simulink model "mmc_model"  (R2023b)
settings: Solver=VariableStepAuto  StartTime=0.0  StopTime=simulation.tsim  RelTol=1e-3
values from neighbouring files (symbols this model uses):
  ab0_to_cell = inv(cell_to_2ab0)    [init_mmc.m]
  cell_to_2ab0 = kron(abc_to_ab0, abc_to_ab0)    [init_mmc.m]
  grid_to_cell = kron(eye(3), ones(3, 1))    [init_mmc.m]
  J = [0 -1; 1 0]    [init_mmc.m]
  machine_to_cell = kron(ones(3, 1), eye(3))    [init_mmc.m]
  volt_to_cell = [      [          1 0 0 0 0 0 ... (first row only)    [init_mmc.m]
undefined symbols (not defined in the file or in its folder): avi, clc, cpu, ctrl, currentControl, DiscIntNeverNeededParam, gfl, grid, load2, loadStep, machine, mmc, pq_ctrl, simulation, soa, stiffGrid, sync, testScenario
libraries: library x17, spsThreePhaseSeriesRLCBranchLib x16, eeGeneralControl x15, spsControlledVoltageSourceLib x15, simulink x11, spsThreePhaseVIMeasurementLib x10, spsGroundLib x9, eeDiscretePi x8, simulink_extras x8, spsabctodq0Lib x8, spsThreePhaseBreakerLib x7, spsdq0toabcLib x5
(part 2 of 3)

== system mmc_model/Electrical Model/Variant Subsystem ==
  note: 1) Add Subsystem or Model blocks as valid variant choices.
      | 2) You cannot connect blocks at this level. At simulation, connectivity is automatically
      | determined, based on the active variant and port name matching.
  GFL_VSC : Subsystem  VariantControl=machine.grid==2
  GFL_VSC_noDC : Subsystem  VariantControl=machine.grid==4
  infinite_bus : Subsystem  VariantControl=machine.grid==0
  short_circuited : Subsystem  VariantControl=machine.grid==3
  synchronous_machine : Subsystem  VariantControl=machine.grid==1
  A : PMIOPort  Side=Left
  B : PMIOPort  Port=2  Side=Left
  C : PMIOPort  Port=3  Side=Left

== system mmc_model/dq_to_ab_g/Subsystem ==
  dq : Inport  PortDimensions=2
  wt : Inport  Port=2  PortDimensions=1
  Fcn : Fcn  Expr=u[1]*cos(u[3]) - u[2]*sin(u[3])
  Fcn1 : Fcn  Expr=u[1]*sin(u[3]) + u[2]*cos(u[3])
  Mux11 : Mux  Inputs=2
  Mux12 : Mux  Inputs=[2 1]
  Mux13 : Mux  Inputs=[2 1]
  alpha_beta : Outport  InitialOutput=[0,0]  VectorParamsAs1DForOutWhenUnconnected=off
  wires:
  wt/1 -> Mux13/2, Mux12/2
  Fcn1/1 -> Mux11/2
  Mux11/1 -> alpha_beta/1
  dq/1 -> Mux13/1, Mux12/1
  Fcn/1 -> Mux11/1
  Mux12/1 -> Fcn/1
  Mux13/1 -> Fcn1/1

== system mmc_model/dq_to_ab_g/Subsystem1 ==
  dq : Inport  PortDimensions=2
  wt : Inport  Port=2  PortDimensions=1
  Fcn : Fcn  Expr=u[1]*cos(u[3]) - u[2]*sin(u[3])
  Fcn1 : Fcn  Expr=u[1]*sin(u[3]) + u[2]*cos(u[3])
  Mux11 : Mux  Inputs=2
  Mux12 : Mux  Inputs=[2 1]
  Mux13 : Mux  Inputs=[2 1]
  alpha_beta : Outport  InitialOutput=[0,0]  VectorParamsAs1DForOutWhenUnconnected=off
  wires:
  wt/1 -> Mux13/2, Mux12/2
  Fcn1/1 -> Mux11/2
  Mux11/1 -> alpha_beta/1
  dq/1 -> Mux13/1, Mux12/1
  Fcn/1 -> Mux11/1
  Mux12/1 -> Fcn/1
  Mux13/1 -> Fcn1/1

== system mmc_model/dq_to_ab_m/Subsystem ==
  dq : Inport  PortDimensions=2
  wt : Inport  Port=2  PortDimensions=1
  Fcn : Fcn  Expr=u[1]*cos(u[3]) - u[2]*sin(u[3])
  Fcn1 : Fcn  Expr=u[1]*sin(u[3]) + u[2]*cos(u[3])
  Mux11 : Mux  Inputs=2
  Mux12 : Mux  Inputs=[2 1]
  Mux13 : Mux  Inputs=[2 1]
  alpha_beta : Outport  InitialOutput=[0,0]  VectorParamsAs1DForOutWhenUnconnected=off
  wires:
  wt/1 -> Mux13/2, Mux12/2
  Fcn1/1 -> Mux11/2
  Mux11/1 -> alpha_beta/1
  dq/1 -> Mux13/1, Mux12/1
  Fcn/1 -> Mux11/1
  Mux12/1 -> Fcn/1
  Mux13/1 -> Fcn1/1

== system mmc_model/dq_to_ab_m/Subsystem1 ==
  dq : Inport  PortDimensions=2
  wt : Inport  Port=2  PortDimensions=1
  Fcn : Fcn  Expr=u[1]*cos(u[3]) - u[2]*sin(u[3])
  Fcn1 : Fcn  Expr=u[1]*sin(u[3]) + u[2]*cos(u[3])
  Mux11 : Mux  Inputs=2
  Mux12 : Mux  Inputs=[2 1]
  Mux13 : Mux  Inputs=[2 1]
  alpha_beta : Outport  InitialOutput=[0,0]  VectorParamsAs1DForOutWhenUnconnected=off
  wires:
  wt/1 -> Mux13/2, Mux12/2
  Fcn1/1 -> Mux11/2
  Mux11/1 -> alpha_beta/1
  dq/1 -> Mux13/1, Mux12/1
  Fcn/1 -> Mux11/1
  Mux12/1 -> Fcn/1
  Mux13/1 -> Fcn1/1

== system mmc_model/dq_to_ab_ns/Subsystem ==
  dq : Inport  PortDimensions=2
  wt : Inport  Port=2  PortDimensions=1
  Fcn : Fcn  Expr=u[1]*cos(u[3]) - u[2]*sin(u[3])
  Fcn1 : Fcn  Expr=u[1]*sin(u[3]) + u[2]*cos(u[3])
  Mux11 : Mux  Inputs=2
  Mux12 : Mux  Inputs=[2 1]
  Mux13 : Mux  Inputs=[2 1]
  alpha_beta : Outport  InitialOutput=[0,0]  VectorParamsAs1DForOutWhenUnconnected=off
  wires:
  wt/1 -> Mux13/2, Mux12/2
  Fcn1/1 -> Mux11/2
  Mux11/1 -> alpha_beta/1
  dq/1 -> Mux13/1, Mux12/1
  Fcn/1 -> Mux11/1
  Mux12/1 -> Fcn/1
  Mux13/1 -> Fcn1/1

== system mmc_model/dq_to_ab_ns/Subsystem1 ==
  dq : Inport  PortDimensions=2
  wt : Inport  Port=2  PortDimensions=1
  Fcn : Fcn  Expr=u[1]*cos(u[3]) - u[2]*sin(u[3])
  Fcn1 : Fcn  Expr=u[1]*sin(u[3]) + u[2]*cos(u[3])
  Mux11 : Mux  Inputs=2
  Mux12 : Mux  Inputs=[2 1]
  Mux13 : Mux  Inputs=[2 1]
  alpha_beta : Outport  InitialOutput=[0,0]  VectorParamsAs1DForOutWhenUnconnected=off
  wires:
  wt/1 -> Mux13/2, Mux12/2
  Fcn1/1 -> Mux11/2
  Mux11/1 -> alpha_beta/1
  dq/1 -> Mux13/1, Mux12/1
  Fcn/1 -> Mux11/1
  Mux12/1 -> Fcn/1
  Mux13/1 -> Fcn1/1

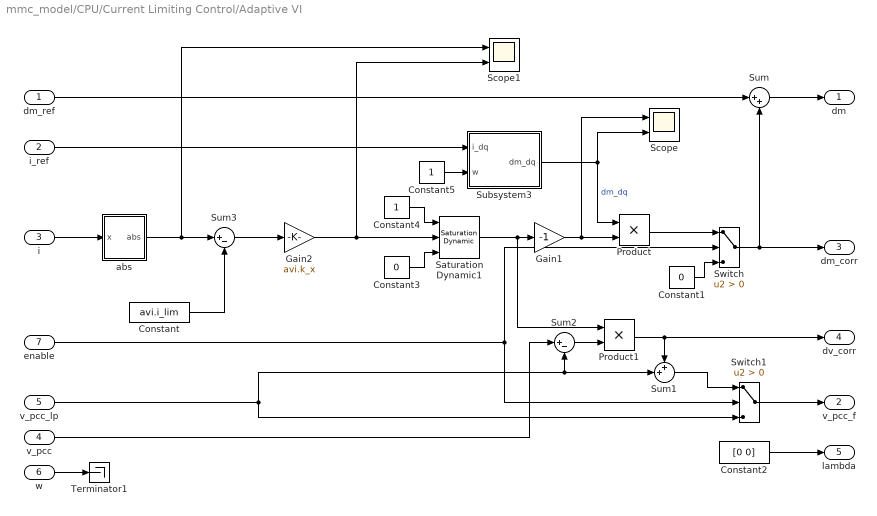
== system mmc_model/CPU/Current Limiting Control/Adaptive VI ==
  dm_ref : Inport
  i_ref : Inport  Port=2
  i : Inport  Port=3
  v_pcc : Inport  Port=4
  v_pcc_lp : Inport  Port=5
  w : Inport  Port=6
  enable : Inport  Port=7
  Constant : Constant  Value=avi.i_lim
  Constant1 : Constant  Value=0
  Constant2 : Constant  Value=[0 0]
  Constant3 : Constant  Value=0
  Constant4 : Constant
  Constant5 : Constant
  Gain1 : Gain  Gain=-1
  Gain2 : Gain  Gain=avi.k_x
  Product : Product
  Product1 : Product
  Saturation Dynamic1 : simulink/Discontinuities/Saturation Dynamic  OutMin=[]  OutMax=[]  OutDataTypeStr=Inherit: Same as second input  OutDataType=fixdt(1, 16)  OutScaling=2^-10  DoSatur=off
  Scope : Scope  NumInputPorts=2
  Scope1 : Scope  NumInputPorts=2
  Subsystem3 : Subsystem
  Sum : Sum  Inputs=|++
  Sum1 : Sum  Inputs=++|
  Sum2 : Sum  Inputs=|+-
  Sum3 : Sum  Inputs=|+-
  Switch : Switch  Criteria=u2 > Threshold  SaturateOnIntegerOverflow=off  InputSameDT=off
  Switch1 : Switch  Criteria=u2 > Threshold  SaturateOnIntegerOverflow=off  InputSameDT=off
  Terminator1 : Terminator
  abs : Subsystem
  dm : Outport
  v_pcc_f : Outport  Port=2
  dm_corr : Outport  Port=3
  dv_corr : Outport  Port=4
  lambda : Outport  Port=5
  wires:
  i/1 -> abs/1(x)
  v_pcc/1 -> Sum2/1
  w/1 -> Terminator1/1
  Constant2/1 -> lambda/1
  Constant/1 -> Sum3/2
  Sum3/1 -> Gain2/1
  abs/1(abs) -> Sum3/1, Scope1/1
  i_ref/1 -> Subsystem3/1(i_dq)
  Subsystem3/1(dm_dq) -> Product/1, Scope/2  "dm_dq"
  dm_ref/1 -> Sum/1
  Sum/1 -> dm/1
  Switch/1 -> Sum/2, dm_corr/1
  enable/1 -> Switch1/2, Switch/2
  Product/1 -> Switch/1
  v_pcc_lp/1 -> Sum2/2, Sum1/2, Switch1/3
  Constant1/1 -> Switch/3
  Constant3/1 -> Saturation Dynamic1/3
  Constant4/1 -> Saturation Dynamic1/1
  Gain2/1 -> Scope1/2, Saturation Dynamic1/2
  Constant5/1 -> Subsystem3/2(w)
  Saturation Dynamic1/1 -> Product1/1, Gain1/1
  Gain1/1 -> Scope/1, Product/2
  Product1/1 -> dv_corr/1, Sum1/1
  Sum1/1 -> Switch1/1
  Sum2/1 -> Product1/2
  Switch1/1 -> v_pcc_f/1

== system mmc_model/CPU/Current Limiting Control/Current Control ==
  dm_ref : Inport
  i_ref : Inport  Port=2
  i : Inport  Port=3
  v_pcc_lp : Inport  Port=4
  enable : Inport  Port=5
  Constant : Constant  Value=currentControl.i_lim
  Constant15 : Constant  Value=0
  Constant2 : Constant  Value=[0 0]
  Logical Operator : Logic  AllPortsSameDT=off  OutDataTypeStr=boolean
  Relay : Relay  OnSwitchValue=0  OffSwitchValue=-0.03
  Scope : Scope  NumInputPorts=2
  Scope1 : Scope
  Sum2 : Sum  Inputs=++|
  Sum3 : Sum  Inputs=|+-
  abs : Subsystem
  iM Control : library/PI Controller  VariantControl=overcurr_ctrl.sel==1  kp=ctrl.machine.ictrl.kp  ti=ctrl.machine.ictrl.ti  Kaw=1
  dm : Outport
  v_pcc_f : Outport  Port=2
  dm_corr : Outport  Port=3
  dv_corr : Outport  Port=4
  lambda : Outport  Port=5
  wires:
  i/1 -> Scope1/1, abs/1(x), iM Control/2
  Constant15/1 -> iM Control/3
  dm_ref/1 -> Sum2/1
  enable/1 -> Logical Operator/2
  Sum2/1 -> dm/1  "dv_m"
  i_ref/1 -> iM Control/1
  iM Control/1 -> dm_corr/1, Sum2/2
  Constant2/1 -> lambda/1, dv_corr/1
  v_pcc_lp/1 -> v_pcc_f/1
  abs/1(abs) -> Sum3/1
  Constant/1 -> Sum3/2
  Relay/1 -> Scope/2, Logical Operator/1
  Logical Operator/1 -> iM Control/4
  Sum3/1 -> Scope/1, Relay/1

== system mmc_model/CPU/Current Limiting Control/Current Limiting Control ==
  dm_ref : Inport
  i_ref : Inport  Port=2
  i : Inport  Port=3
  v_pcc_lp : Inport  Port=4
  w : Inport  Port=5
  enable : Inport  Port=6
  Constant2 : Constant  Value=[0 0]
  Gain : Gain  Gain=1/clc.k_pcc
  Gain1 : Gain  Gain=clc.k_pcc
  Product1 : Product
  SOA_iref : Subsystem
  Scope : Scope  Commented=on  NumInputPorts=3
  Subsystem3 : Subsystem
  Sum2 : Sum  Inputs=|+-
  Sum3 : Sum  Inputs=|-+
  Sum4 : Sum  Inputs=|+-
  Sum5 : Sum  Inputs=|++
  Sum6 : Sum  Inputs=|++
  Terminator1 : Terminator
  dm : Outport
  v_pcc_f : Outport  Port=2
  dm_corr : Outport  Port=3
  dv_corr : Outport  Port=4
  lambda : Outport  Port=5
  wires:
  Constant2/1 -> dv_corr/1, lambda/1
  i/1 -> Sum4/2, Sum5/2, Subsystem3/1(i_dq)
  Sum3/1 -> dm_corr/1
  v_pcc_lp/1 -> v_pcc_f/1
  w/1 -> Subsystem3/2(w)
  Subsystem3/1(dm_dq) -> Sum6/2, Sum2/2  "dm_dq"
  Product1/1 -> Sum3/2, dm/1
  dm_ref/1 -> Sum3/1, Sum2/1
  enable/1 -> Product1/2
  i_ref/1 -> Scope/3
  Sum2/1 -> Gain/1
  Gain/1 -> Sum5/1
  Sum5/1 -> Scope/2, SOA_iref/1(i_ref_dq)
  SOA_iref/1(i_ref_dq_lim) -> Scope/1, Sum4/1  "i_ref_dq"
  Sum4/1 -> Gain1/1
  Gain1/1 -> Sum6/1
  Sum6/1 -> Product1/1

== system mmc_model/CPU/Current Limiting Control/Open Loop ==
  dm_ref : Inport
  v_pcc_lp : Inport  Port=2
  Constant1 : Constant  Value=[0 0]
  dm : Outport
  v_pcc_f : Outport  Port=2
  dm_corr : Outport  Port=3
  dv_corr : Outport  Port=4
  lambda : Outport  Port=5
  wires:
  dm_ref/1 -> dm/1  "dv_m"
  v_pcc_lp/1 -> v_pcc_f/1
  Constant1/1 -> lambda/1, dv_corr/1, dm_corr/1

== system mmc_model/CPU/Current Limiting Control/Safety Filter ==
  dm_ref : Inport
  i_ref : Inport  Port=2
  i : Inport  Port=3
  v_pcc : Inport  Port=4
  enable : Inport  Port=5
  i0 : Inport  Port=6
  v_pcc_lp : Inport  Port=7
  MATLAB Function : MATLAB Function  TreatAsAtomicUnit=on
  Mux : Mux  Inputs=[2 2 2 2 1 1]
  Reshape{,1..3} (4 alike) : Reshape  OutputDimensionality=Customize  OutputDimensions=[2,1]
  Reshape4 : Reshape  OutputDimensionality=Customize  OutputDimensions=[2]
  Reshape5 : Reshape  OutputDimensionality=Customize  OutputDimensions=[2]
  Reshape8 : Reshape  OutputDimensionality=Customize  OutputDimensions=[2]
  Sum : Sum  Inputs=|-+
  correction : Subsystem
  dm : Outport
  v_pcc_f : Outport  Port=2
  dm_corr : Outport  Port=3
  lambda : Outport  Port=4
  wires:
  Reshape1/1 -> Mux/2
  Reshape5/1 -> dm_corr/1
  enable/1 -> Mux/5
  MATLAB Function/2(dm_corr) -> Reshape5/1
  MATLAB Function/1(dm) -> Reshape4/1
  Reshape2/1 -> Mux/3
  dm_ref/1 -> Reshape/1
  Reshape/1 -> Mux/1
  i/1 -> Reshape2/1
  Reshape3/1 -> Mux/4
  Mux/1 -> MATLAB Function/1(u)
  Reshape8/1 -> lambda/1
  MATLAB Function/3(lambda) -> Reshape8/1
  i_ref/1 -> Reshape1/1
  i0/1 -> Mux/6
  Sum/1 -> Reshape3/1
  v_pcc_lp/1 -> v_pcc_f/1, Sum/2
  Reshape4/1 -> dm/1
  v_pcc/1 -> Sum/1

== system mmc_model/CPU/Current Limiting Control/Safety Filter B only ==
  dm_ref : Inport
  i_ref : Inport  Port=2
  i : Inport  Port=3
  v_pcc : Inport  Port=4
  enable : Inport  Port=5
  i0 : Inport  Port=6
  v_pcc_lp : Inport  Port=7
  MATLAB Function : MATLAB Function  TreatAsAtomicUnit=on
  Mux : Mux  Inputs=[2 2 2 2 1 1]
  Reshape{,1..3} (4 alike) : Reshape  OutputDimensionality=Customize  OutputDimensions=[2,1]
  Reshape4 : Reshape  OutputDimensionality=Customize  OutputDimensions=[2]
  Reshape5 : Reshape  OutputDimensionality=Customize  OutputDimensions=[2]
  Reshape8 : Reshape  OutputDimensionality=Customize  OutputDimensions=[2]
  Sum : Sum  Inputs=|-+
  dm : Outport
  v_pcc_f : Outport  Port=2
  dm_corr : Outport  Port=3
  lambda : Outport  Port=4
  wires:
  Reshape1/1 -> Mux/2
  Reshape5/1 -> dm_corr/1
  enable/1 -> Mux/5
  MATLAB Function/2(dm_corr) -> Reshape5/1
  MATLAB Function/1(dm) -> Reshape4/1
  Reshape2/1 -> Mux/3
  dm_ref/1 -> Reshape/1
  Reshape/1 -> Mux/1
  i/1 -> Reshape2/1
  Reshape3/1 -> Mux/4
  Mux/1 -> MATLAB Function/1(u)
  Reshape8/1 -> lambda/1
  MATLAB Function/3(lambda) -> Reshape8/1
  i_ref/1 -> Reshape1/1
  i0/1 -> Mux/6
  Sum/1 -> Reshape3/1
  v_pcc/1 -> Sum/1
  v_pcc_lp/1 -> v_pcc_f/1, Sum/2
  Reshape4/1 -> dm/1

== system mmc_model/CPU/GFM Control/EDPC ==
  pq_ref : Inport
  pq : Inport  Port=2
  v_pcc_abs : Inport  Port=3
  antiwindup : Inport  Port=4
  enable : Inport  Port=5
  Complex to Real-Imag : ComplexToRealImag
  Constant : Constant
  Demux2 : Demux  Outputs=2
  Demux3 : Demux  Outputs=2
  Magnitude-Angle to Complex : MagnitudeAngleToComplex
  Mux1 : Mux  Inputs=2
  NOT1 : Logic  Operator=NOT  IconShape=distinctive  AllPortsSameDT=off  OutDataTypeStr=boolean
  PCtrl : eeDiscretePi/Discrete PI Controller  Kp=pq_ctrl.kp*machine.tr.l  Ki=pq_ctrl.ki*machine.tr.l  Kaw=1000  x0=0  Ts=-1
      settings: LibrarySourceBlock=ee_sl_lib/General Control/Discrete PI Controller
  Product1 : Product
  Product2 : Product
  QCtrl : eeDiscretePi/Discrete PI Controller  Kp=pq_ctrl.kp  Ki=pq_ctrl.ki  Kaw=1000  x0=0  Ts=-1
      settings: LibrarySourceBlock=ee_sl_lib/General Control/Discrete PI Controller
  Saturation : Saturate  UpperLimit=pi/3  LowerLimit=-pi/3
  Scope : Scope  Commented=on
  Sum : Sum  Inputs=|++
  Sum1 : Sum  Inputs=-|+
  Sum2 : Sum  Inputs=|++
  Sum4 : Sum  Inputs=|+-
  abs_phi1 : Scope  Commented=on  NumInputPorts=2
  uQ Droop2 : Gain  Gain=-1
  m : Outport
  wires:
  Sum4/1 -> Demux3/1
  NOT1/1 -> QCtrl/3, PCtrl/3
  pq/1 -> Sum4/2
  Magnitude-Angle to Complex/1 -> Complex to Real-Imag/1
  Complex to Real-Imag/1 -> Mux1/1
  Complex to Real-Imag/2 -> Mux1/2
  Sum2/1 -> Magnitude-Angle to Complex/1
  Product2/1 -> Magnitude-Angle to Complex/2
  Constant/1 -> Sum2/2
  enable/1 -> Product2/1, Product1/1, NOT1/1
  Mux1/1 -> m/1
  antiwindup/1 -> Demux2/1
  PCtrl/1 -> Sum1/1, Saturation/1
  Product1/1 -> Sum2/1
  Demux3/1 -> PCtrl/1
  pq_ref/1 -> Sum4/1
  Demux3/2 -> QCtrl/1
  Saturation/1 -> Sum1/2, abs_phi1/1, Product2/2
  QCtrl/1 -> uQ Droop2/1
  uQ Droop2/1 -> Product1/2, abs_phi1/2
  v_pcc_abs/1 -> Scope/1
  Demux2/2 -> QCtrl/2
  Demux2/1 -> Sum/1
  Sum1/1 -> Sum/2
  Sum/1 -> PCtrl/2

== system mmc_model/CPU/GFM Control/EDPC (modified) ==
  pq_ref : Inport
  pq : Inport  Port=2
  w : Inport  Port=3
  v_pcc_lp : Inport  Port=4
  antiwindup : Inport  Port=5
  enable : Inport  Port=6
  NOT1 : Logic  Operator=NOT  IconShape=distinctive  AllPortsSameDT=off  OutDataTypeStr=boolean
  PQCtrl : eeDiscretePi/Discrete PI Controller  Kp=pq_ctrl.kp  Ki=pq_ctrl.ki  Kaw=1000  x0=0  Ts=-1
      settings: LibrarySourceBlock=ee_sl_lib/General Control/Discrete PI Controller
  Product1 : Product
  Sum2 : Sum  Inputs=|++
  Sum4 : Sum  Inputs=|+-
  Z : Subsystem
  m : Outport
  wires:
  PQCtrl/1 -> Product1/1  "i_ref_dq"
  pq_ref/1 -> Sum4/1  "PQ_ref"
  Sum4/1 -> PQCtrl/1
  NOT1/1 -> PQCtrl/3
  enable/1 -> [enable]
  [enable] -> NOT1/1
  [enable] -> Product1/2
  pq/1 -> Sum4/2
  [w] -> Z/2(w)
  Z/1(dm_dq) -> Sum2/1  "dv_m_ref"
  Product1/1 -> Z/1(i_dq)  "i_ref_dq"
  antiwindup/1 -> PQCtrl/2
  v_pcc_lp/1 -> Sum2/2
  Sum2/1 -> m/1
  w/1 -> [w]

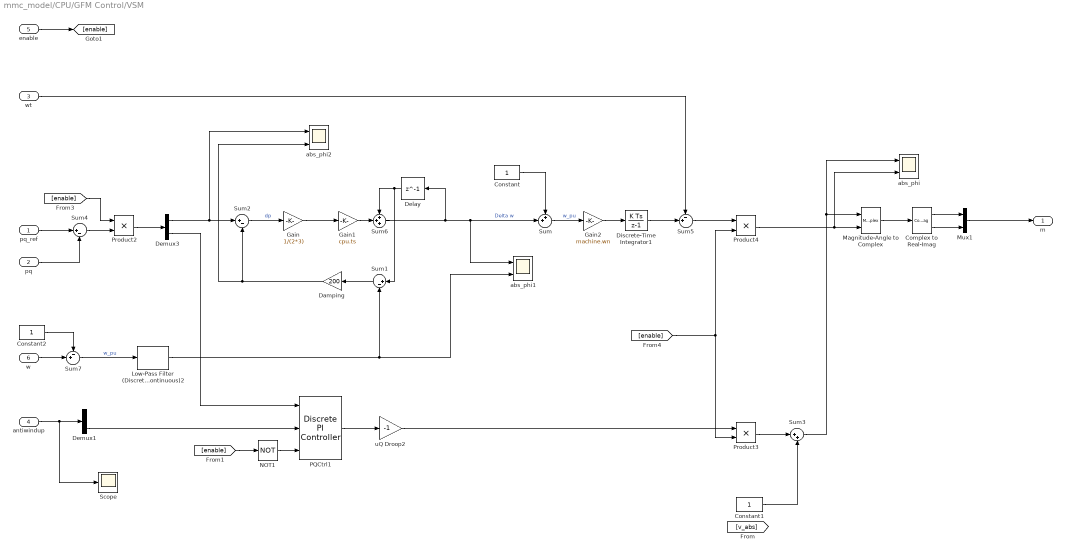
== system mmc_model/CPU/GFM Control/VSM ==
  pq_ref : Inport
  pq : Inport  Port=2
  wt : Inport  Port=3
  antiwindup : Inport  Port=4
  enable : Inport  Port=5
  w : Inport  Port=6
  Complex to Real-Imag : ComplexToRealImag
  Constant : Constant
  Constant1 : Constant
  Constant2 : Constant
  Damping : Gain  Gain=200
  Delay : Delay  DelayLength=1  InitialCondition=0
  Demux1 : Demux  Outputs=2
  Demux3 : Demux  Outputs=2
  Discrete-Time Integrator1 : DiscreteIntegrator  SampleTime=-1  ICPrevOutput=DiscIntNeverNeededParam  ICPrevScaledInput=DiscIntNeverNeededParam
  Gain : Gain  Gain=1/(2*3)
  Gain1 : Gain  Gain=cpu.ts
  Gain2 : Gain  Gain=machine.wn
  Low-Pass Filter (Discrete or Continuous)2 : eeGeneralControl/Low-Pass Filter (Discrete or Continuous)  K=1  T=0.1  B=inf  A=-inf  init_option=Inherited from block input  x0=0  Ts=-1
  Magnitude-Angle to Complex : MagnitudeAngleToComplex
  Mux1 : Mux  Inputs=2
  NOT1 : Logic  Operator=NOT  IconShape=distinctive  AllPortsSameDT=off  OutDataTypeStr=boolean
  PQCtrl1 : eeDiscretePi/Discrete PI Controller  Kp=pq_ctrl.kp  Ki=pq_ctrl.ki  Kaw=1000  x0=0  Ts=-1
      settings: LibrarySourceBlock=ee_sl_lib/General Control/Discrete PI Controller
  Product2 : Product
  Product3 : Product
  Product4 : Product
  Scope : Scope
  Sum : Sum  Inputs=++|
  Sum1 : Sum  Inputs=|+-
  Sum2 : Sum  Inputs=|+-
  Sum3 : Sum  Inputs=|++
  Sum4 : Sum  Inputs=|+-
  Sum5 : Sum  Inputs=-+|
  Sum6 : Sum  Inputs=+++
  Sum7 : Sum  Inputs=-+|
  abs_phi : Scope  NumInputPorts=2
  abs_phi1 : Scope  NumInputPorts=2
  abs_phi2 : Scope  NumInputPorts=2
  uQ Droop2 : Gain  Gain=-1
  m : Outport
  wires:
  Demux3/1 -> abs_phi2/1, Sum2/1
  enable/1 -> [enable]
  Constant/1 -> Sum/1
  Sum1/1 -> Damping/1
  Gain2/1 -> Discrete-Time Integrator1/1
  Sum/1 -> Gain2/1  "w_pu"
  pq/1 -> Sum4/2
  Product2/1 -> Demux3/1
  antiwindup/1 -> Scope/1, Demux1/1
  Demux3/2 -> PQCtrl1/1
  [enable] -> NOT1/1
  NOT1/1 -> PQCtrl1/3
  PQCtrl1/1 -> uQ Droop2/1
  Product3/1 -> Sum3/1
  Sum3/1 -> Magnitude-Angle to Complex/1, abs_phi/1
  Complex to Real-Imag/2 -> Mux1/2
  Magnitude-Angle to Complex/1 -> Complex to Real-Imag/1
  Complex to Real-Imag/1 -> Mux1/1
  Mux1/1 -> m/1
  [enable] -> Product2/1
  wt/1 -> Sum5/1
  Discrete-Time Integrator1/1 -> Sum5/2
  Product4/1 -> abs_phi/2, Magnitude-Angle to Complex/2
  [enable] -> Product4/2, Product3/2
  uQ Droop2/1 -> Product3/1
  Sum5/1 -> Product4/1
  Demux1/2 -> PQCtrl1/2
  Constant1/1 -> Sum3/2
  pq_ref/1 -> Sum4/1
  Sum4/1 -> Product2/2
  Gain1/1 -> Sum6/2
  Delay/1 -> Sum1/1, Sum6/1
  Sum6/1 -> abs_phi1/1, Sum/2, Delay/1  "Delta w"
  Gain/1 -> Gain1/1
  Damping/1 -> abs_phi2/2, Sum2/2
  w/1 -> Sum7/2
  Sum7/1 -> Low-Pass Filter (Discrete or Continuous)2/1  "w_pu"
  Constant2/1 -> Sum7/1
  Sum2/1 -> Gain/1  "dp"
  Low-Pass Filter (Discrete or Continuous)2/1 -> Sum1/2, abs_phi1/2

== system mmc_model/CPU/SOA/SOA_iref ==
  i_ref_dq : Inport
  i_lim_corr : Inport  Port=2
  Constant6 : Constant  Value=soa.i_lim
  Constant7 : Constant  Value=soa.i_lim
  Demux : Demux  Outputs=2
  Gain7 : Gain  Gain=-1
  Gain9 : Gain  Gain=-1
  Mux : Mux  Inputs=2
  Saturation Dynamic1 : simulink/Discontinuities/Saturation Dynamic  OutMin=[]  OutMax=[]  OutDataTypeStr=Inherit: Same as second input  OutDataType=fixdt(1, 16)  OutScaling=2^-10  DoSatur=off
  Saturation Dynamic2 : simulink/Discontinuities/Saturation Dynamic  OutMin=[]  OutMax=[]  OutDataTypeStr=Inherit: Same as second input  OutDataType=fixdt(1, 16)  OutScaling=2^-10  DoSatur=off
  Sqrt3 : Sqrt
  Square1 : Math  Operator=square
  Square4 : Math  Operator=square
  Sum : Sum  Inputs=-+|
  Sum5 : Sum  Inputs=|-+
  i_ref_dq_lim : Outport
  wires:
  Saturation Dynamic1/1 -> Mux/1, Square4/1
  Sqrt3/1 -> Gain7/1, Saturation Dynamic2/1
  Demux/1 -> Saturation Dynamic1/2
  Square4/1 -> Sum5/1
  Sum5/1 -> Sqrt3/1
  Gain7/1 -> Saturation Dynamic2/3
  i_ref_dq/1 -> Demux/1
  Saturation Dynamic2/1 -> Mux/2  "i_q_ref_soa"
  Mux/1 -> i_ref_dq_lim/1
  Square1/1 -> Sum5/2
  Constant6/1 -> Square1/1
  Gain9/1 -> Saturation Dynamic1/3
  Sum/1 -> Saturation Dynamic1/1, Gain9/1
  Constant7/1 -> Sum/2
  i_lim_corr/1 -> Sum/1
  Demux/2 -> Saturation Dynamic2/2

== system mmc_model/CPU/SOA/Subsystem ==
  In1 : Inport
  i_lim_corr : Inport  Port=2
  Cartesian to Polar1 : simulink_extras/Transformations/Cartesian to Polar
  Constant7 : Constant  Value=soa.i_lim
  Demux1 : Demux  Outputs=2
  Gain1 : Gain  Gain=-1
  Mux1 : Mux  Inputs=2
  Polar to Cartesian1 : simulink_extras/Transformations/Polar to Cartesian
  Saturation : Saturate  UpperLimit=inf  LowerLimit=0
  Saturation Dynamic2 : simulink/Discontinuities/Saturation Dynamic  OutMin=[]  OutMax=[]  OutDataTypeStr=Inherit: Same as second input  OutDataType=fixdt(1, 16)  OutScaling=2^-10  DoSatur=off
  Sum : Sum  Inputs=-+|
  Out1 : Outport
  wires:
  Polar to Cartesian1/2 -> Mux1/2
  In1/1 -> Demux1/1
  Gain1/1 -> Saturation Dynamic2/3
  Demux1/1 -> Cartesian to Polar1/1
  Cartesian to Polar1/1 -> Saturation Dynamic2/2
  Sum/1 -> Saturation/1
  Saturation Dynamic2/1 -> Polar to Cartesian1/1
  Demux1/2 -> Cartesian to Polar1/2
  Polar to Cartesian1/1 -> Mux1/1
  Cartesian to Polar1/2 -> Polar to Cartesian1/2
  Mux1/1 -> Out1/1
  i_lim_corr/1 -> Sum/1
  Constant7/1 -> Sum/2
  Saturation/1 -> Gain1/1, Saturation Dynamic2/1

== system mmc_model/CPU/SOA/Subsystem3 ==
  i_dq : Inport
  w : Inport  Port=2
  Gain : Gain  Gain=J  Multiplication=Matrix(K*u) (u vector)
  Gain1 : Gain  Gain=machine.tr.l
  Gain2 : Gain  Gain=machine.tr.r
  Product : Product
  Sum8 : Sum  Inputs=++|
  dm_dq : Outport
  wires:
  Gain1/1 -> Sum8/2
  Sum8/1 -> dm_dq/1  "dm_dq"
  Product/1 -> Gain/1
  Gain/1 -> Gain1/1  "dm_dq"
  w/1 -> Product/1
  i_dq/1 -> Gain2/1, Product/2
  Gain2/1 -> Sum8/1

== system mmc_model/CPU/SOA/Subsystem4 ==
  x : Inport
  y : Inport  Port=2
  Demux : Demux  Outputs=2
  Demux1 : Demux  Outputs=2
  Mux1 : Mux  Inputs=2
  Mux2 : Mux  Inputs=2
  d : Outport
  q : Outport  Port=2
  wires:
  Mux2/1 -> q/1
  y/1 -> Demux1/1
  Demux/2 -> Mux2/1
  Demux1/2 -> Mux2/2
  Demux/1 -> Mux1/1
  Demux1/1 -> Mux1/2
  Mux1/1 -> d/1
  x/1 -> Demux/1

== system mmc_model/CPU/SOA/Z_inv ==
  v : Inport
  w : Inport  Port=2
  Complex to Real-Imag : ComplexToRealImag
  Constant : Constant  Value=machine.tr.r
  Constant1 : Constant  Value=machine.tr.l
  Demux : Demux  Outputs=2
  Divide : Product  Inputs=**
  Divide1 : Product  Inputs=*/
  Mux : Mux  Inputs=2
  Real-Imag to Complex : RealImagToComplex
  Real-Imag to Complex1 : RealImagToComplex
  i : Outport
  wires:
  Real-Imag to Complex1/1 -> Divide1/1
  Complex to Real-Imag/2 -> Mux/2
  Constant/1 -> Real-Imag to Complex/1
  Divide/1 -> Real-Imag to Complex/2
  Demux/2 -> Real-Imag to Complex1/2
  Real-Imag to Complex/1 -> Divide1/2
  Divide1/1 -> Complex to Real-Imag/1
  Constant1/1 -> Divide/1
  Complex to Real-Imag/1 -> Mux/1
  Demux/1 -> Real-Imag to Complex1/1
  w/1 -> Divide/2
  Mux/1 -> i/1
  v/1 -> Demux/1

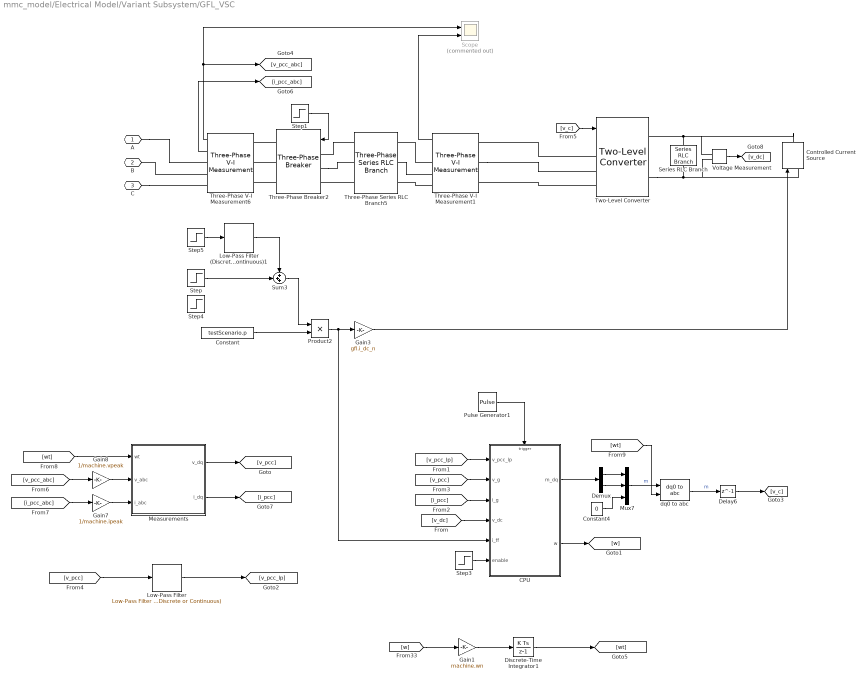
== system mmc_model/Electrical Model/Variant Subsystem/GFL_VSC ==
  CPU : Subsystem
  Constant : Constant  Value=testScenario.p
  Constant4 : Constant  Value=0
  Controlled Current Source : spsControlledCurrentSourceLib/Controlled Current Source  Initialize=on  Source_Type=AC  Amplitude=0  Phase=0  Frequency=0  Measurements=None
  Delay6 : Delay  DelayLength=1  InitialCondition=0  SampleTime=simulation.ts
  Demux : Demux  Outputs=2
  Discrete-Time Integrator1 : DiscreteIntegrator  gainval=1  SampleTime=-1  ICPrevOutput=DiscIntNeverNeededParam  ICPrevScaledInput=DiscIntNeverNeededParam
  Gain1 : Gain  Gain=machine.wn
  Gain3 : Gain  Gain=gfl.i_dc_n
  Gain7 : Gain  Gain=1/machine.ipeak
  Gain8 : Gain  Gain=1/machine.vpeak
  Low-Pass Filter : eeGeneralControl/Low-Pass Filter (Discrete or Continuous)  K=1  T=1/machine.wn*10  B=inf  A=-inf  init_option=Specify as parameter  x0=[1 0 0]  Ts=-1
  Low-Pass Filter (Discrete or Continuous)1 : eeGeneralControl/Low-Pass Filter (Discrete or Continuous)  K=1  T=1e-1  B=inf  A=-inf  init_option=Inherited from block input  x0=0  Ts=-1
  Measurements : Subsystem
  Mux7 : Mux  Inputs=3
  Product2 : Product
  Pulse Generator1 : DiscretePulseGenerator  PulseType=Time based  Period=cpu.ts  PulseWidth=50
  Scope : Scope  Commented=on  NumInputPorts=2
  Series RLC Branch : spsSeriesRLCBranchLib/Series RLC Branch  LConnTagsString=__new0  RConnTagsString=__new0  BranchType=C  Resistance=1  Inductance=1e-3  SetiL0=off  InitialCurrent=0  Capacitance=gfl.c_dc_si  Setx0=on  InitialVoltage=gfl.v_dc  Measurements=None
  Step : Step  Time=loadStep.stepDown  After=-1
  Step1 : Step  Time=gfl.breaker_close
  Step3 : Step  Time=ctrl.grid.ictrl.enable
  Step4 : Step  Time=loadStep.stepUp
  Step5 : Step  Time=gfl.ref_step
  Sum3 : Sum  Inputs=+++
  Three-Phase Series RLC Branch5 : spsThreePhaseSeriesRLCBranchLib/Three-Phase Series RLC Branch  LConnTagsString=A|B|C  RConnTagsString=A|B|C  BranchType=RL  Resistance=gfl.tr.r_si  Inductance=gfl.tr.l_si  Capacitance=1e-6  Measurements=None
  Three-Phase V-I Measurement1 : spsThreePhaseVIMeasurementLib/Three-Phase V-I Measurement  VoltageMeasurement=phase-to-ground  SetLabelV=off  LabelV=Vabc  Vpu=off  VpuLL=off  CurrentMeasurement=yes  SetLabelI=off  LabelI=Iabc  Ipu=off  Pbase=100e6  Vbase=500e3  OutputType=Complex  PhasorSimulation=off  PSBequivalent=0
  Three-Phase V-I Measurement6 : spsThreePhaseVIMeasurementLib/Three-Phase V-I Measurement  VoltageMeasurement=phase-to-ground  SetLabelV=off  LabelV=Vabc  Vpu=off  VpuLL=off  CurrentMeasurement=yes  SetLabelI=off  LabelI=Iabc  Ipu=off  Pbase=100e6  Vbase=500e3  OutputType=Complex  PhasorSimulation=off  PSBequivalent=0
  Three-Phase Breaker2 : spsThreePhaseBreakerLib/Three-Phase Breaker  InitialState=open  SwitchA=on  SwitchB=on  SwitchC=on  SwitchTimes=[machine.breaker_close]  External=on  BreakerResistance=0.01  SnubberResistance=1e6  SnubberCapacitance=inf  Measurements=None
  Two-Level Converter : spsTwoLevelConverterLib/Two-Level Converter  ModelType=Average model (Uref-controlled)  Ron=1e-3  Rs=1e6  Cs=inf  Vforward=[0,0]  Ron_Diode=1e-3  Rs_Diode=1e6  Cs_Diode=inf  Vf_Diode=1e-3  Rs_CurrentSource=inf  Ron_ACsource=1e-3
      settings: LibrarySourceBlock=sps_lib/Power Electronics/Two-Level Converter
  Voltage Measurement : spsVoltageMeasurementLib/Voltage Measurement  PhasorSimulation=off  OutputType=Complex  PSBequivalent=0
  dq0 to abc : spsdq0toabcLib/dq0 to abc  Alignment=Aligned with phase A axis
  A : PMIOPort  Side=Left
  B : PMIOPort  Port=2  Side=Left
  C : PMIOPort  Port=3  Side=Left
  wires:
  [v_pcc_abc] -> Gain8/1
  [i_pcc_abc] -> Gain7/1
  [wt] -> Measurements/1(wt)
  Demux/2 -> Mux7/2
  Constant4/1 -> Mux7/3
  Mux7/1 -> dq0 to abc/1  "m"
  Demux/1 -> Mux7/1
  [wt] -> dq0 to abc/2
  CPU/1(m_dq) -> Demux/1
  [i_pcc] -> CPU/3(i_g)
  Pulse Generator1/1 -> CPU/Trigger
  [v_pcc_lp] -> CPU/1(v_pcc_lp)
  Step3/1 -> CPU/6(enable)
  Measurements/2(i_dq) -> [i_pcc]
  Measurements/1(v_dq) -> [v_pcc]
  [v_pcc] -> Low-Pass Filter/1
  Low-Pass Filter/1 -> [v_pcc_lp]
  Gain7/1 -> Measurements/3(i_abc)
  Gain8/1 -> Measurements/2(v_abc)
  CPU/2(w) -> [w]
  [v_pcc] -> CPU/2(v_g)
  [w] -> Gain1/1
  Gain1/1 -> Discrete-Time Integrator1/1
  Discrete-Time Integrator1/1 -> [wt]
  Step1/1 -> Three-Phase Breaker2/1
  Three-Phase V-I Measurement6/1 -> [v_pcc_abc], Scope/1
  Three-Phase V-I Measurement6/2 -> [i_pcc_abc]
  dq0 to abc/1 -> Delay6/1  "m"
  Delay6/1 -> [v_c]
  Voltage Measurement/1 -> [v_dc]
  [v_c] -> Two-Level Converter/1
  [v_dc] -> CPU/4(v_dc)
  Three-Phase V-I Measurement1/1 -> Scope/2
  Low-Pass Filter (Discrete or Continuous)1/1 -> Sum3/1
  Step5/1 -> Low-Pass Filter (Discrete or Continuous)1/1
  Sum3/1 -> Product2/1
  Constant/1 -> Product2/2
  Product2/1 -> CPU/5(i_ff), Gain3/1
  Gain3/1 -> Controlled Current Source/1
  Step/1 -> Sum3/2
  connections:
  Three-Phase Series RLC Branch5/LConn3 -- Three-Phase Breaker2/LConn3
  Three-Phase Breaker2/RConn1 -- Three-Phase V-I Measurement6/LConn1
  Three-Phase Breaker2/RConn2 -- Three-Phase V-I Measurement6/LConn2
  Three-Phase Breaker2/LConn2 -- Three-Phase Series RLC Branch5/LConn2
  Three-Phase Series RLC Branch5/LConn1 -- Three-Phase Breaker2/LConn1
  Three-Phase Breaker2/RConn3 -- Three-Phase V-I Measurement6/LConn3
  A/RConn1 -- Three-Phase V-I Measurement6/RConn1
  Three-Phase V-I Measurement6/RConn2 -- B/RConn1
  C/RConn1 -- Three-Phase V-I Measurement6/RConn3
  Two-Level Converter/LConn1 -- Three-Phase V-I Measurement1/LConn1
  Three-Phase V-I Measurement1/LConn2 -- Two-Level Converter/LConn2
  Two-Level Converter/LConn3 -- Three-Phase V-I Measurement1/LConn3
  Series RLC Branch/LConn1 -- Voltage Measurement/LConn1 -- Controlled Current Source/RConn1 -- Two-Level Converter/RConn1
  Two-Level Converter/RConn2 -- Voltage Measurement/LConn2 -- Controlled Current Source/LConn1 -- Series RLC Branch/RConn1
  Three-Phase V-I Measurement1/RConn1 -- Three-Phase Series RLC Branch5/RConn1
  Three-Phase Series RLC Branch5/RConn2 -- Three-Phase V-I Measurement1/RConn2
  Three-Phase V-I Measurement1/RConn3 -- Three-Phase Series RLC Branch5/RConn3

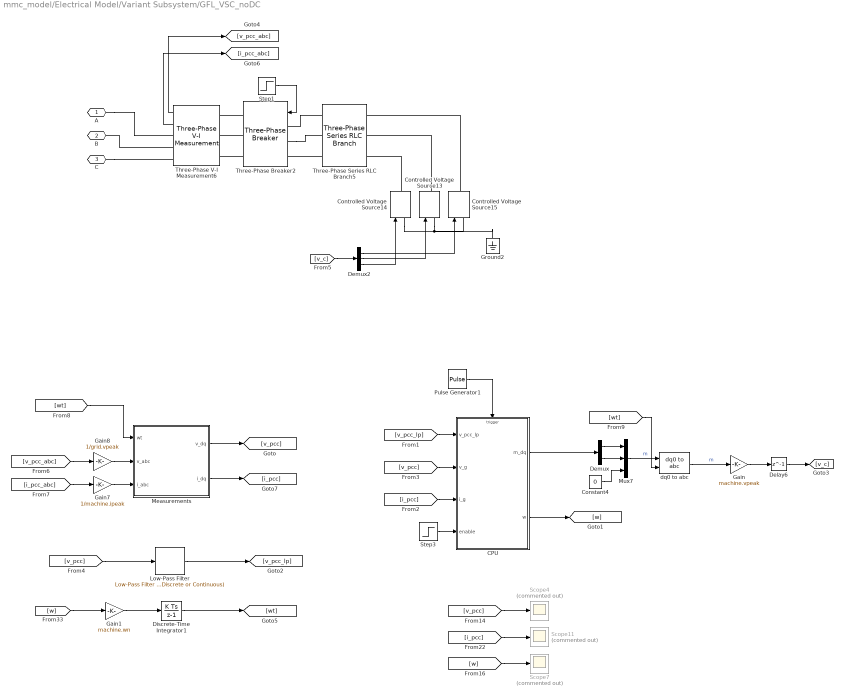
== system mmc_model/Electrical Model/Variant Subsystem/GFL_VSC_noDC ==
  CPU : Subsystem
  Constant4 : Constant  Value=0
  Controlled Voltage Source13 : spsControlledVoltageSourceLib/Controlled Voltage Source  Initialize=on  Source_Type=AC  Amplitude=0  Phase=0  Frequency=0  Measurements=None
  Controlled Voltage Source14 : spsControlledVoltageSourceLib/Controlled Voltage Source  Initialize=on  Source_Type=AC  Amplitude=0  Phase=0  Frequency=0  Measurements=None
  Controlled Voltage Source15 : spsControlledVoltageSourceLib/Controlled Voltage Source  Initialize=on  Source_Type=AC  Amplitude=0  Phase=0  Frequency=0  Measurements=None
  Delay6 : Delay  DelayLength=1  InitialCondition=0  SampleTime=simulation.ts
  Demux : Demux  Outputs=2
  Demux2 : Demux  Outputs=3
  Discrete-Time Integrator1 : DiscreteIntegrator  gainval=1  SampleTime=-1  ICPrevOutput=DiscIntNeverNeededParam  ICPrevScaledInput=DiscIntNeverNeededParam
  Gain : Gain  Gain=machine.vpeak
  Gain1 : Gain  Gain=machine.wn
  Gain7 : Gain  Gain=1/machine.ipeak
  Gain8 : Gain  Gain=1/grid.vpeak
  Ground2 : spsGroundLib/Ground  LConnTagsString=a
  Low-Pass Filter : eeGeneralControl/Low-Pass Filter (Discrete or Continuous)  K=1  T=1/machine.wn*10  B=inf  A=-inf  init_option=Specify as parameter  x0=[1 0 0]  Ts=-1
  Measurements : Subsystem
  Mux7 : Mux  Inputs=3
  Pulse Generator1 : DiscretePulseGenerator  PulseType=Time based  Period=cpu.ts  PulseWidth=50
  Scope11 : Scope  Commented=on
  Scope4 : Scope  Commented=on
  Scope7 : Scope  Commented=on
  Step1 : Step  Time=gfl.breaker_close
  Step3 : Step  Time=gfl.ctrl_enable
  Three-Phase Series RLC Branch5 : spsThreePhaseSeriesRLCBranchLib/Three-Phase Series RLC Branch  LConnTagsString=A|B|C  RConnTagsString=A|B|C  BranchType=RL  Resistance=gfl.tr.r_si  Inductance=gfl.tr.l_si  Capacitance=1e-6  Measurements=None
  Three-Phase V-I Measurement6 : spsThreePhaseVIMeasurementLib/Three-Phase V-I Measurement  VoltageMeasurement=phase-to-ground  SetLabelV=off  LabelV=Vabc  Vpu=off  VpuLL=off  CurrentMeasurement=yes  SetLabelI=off  LabelI=Iabc  Ipu=off  Pbase=100e6  Vbase=500e3  OutputType=Complex  PhasorSimulation=off  PSBequivalent=0
  Three-Phase Breaker2 : spsThreePhaseBreakerLib/Three-Phase Breaker  InitialState=open  SwitchA=on  SwitchB=on  SwitchC=on  SwitchTimes=[machine.breaker_close]  External=on  BreakerResistance=0.01  SnubberResistance=1e6  SnubberCapacitance=inf  Measurements=None
  dq0 to abc : spsdq0toabcLib/dq0 to abc  Alignment=Aligned with phase A axis
  A : PMIOPort  Side=Left
  B : PMIOPort  Port=2  Side=Left
  C : PMIOPort  Port=3  Side=Left
  wires:
  [v_pcc_abc] -> Gain8/1
  [i_pcc_abc] -> Gain7/1
  [wt] -> Measurements/1(wt)
  Demux/2 -> Mux7/2
  Constant4/1 -> Mux7/3
  Mux7/1 -> dq0 to abc/1  "m"
  Demux/1 -> Mux7/1
  [wt] -> dq0 to abc/2
  Gain/1 -> Delay6/1
  CPU/1(m_dq) -> Demux/1
  [i_pcc] -> CPU/3(i_g)
  Pulse Generator1/1 -> CPU/Trigger
  [v_pcc_lp] -> CPU/1(v_pcc_lp)
  Step3/1 -> CPU/4(enable)
  Measurements/2(i_dq) -> [i_pcc]
  Measurements/1(v_dq) -> [v_pcc]
  [v_pcc] -> Low-Pass Filter/1
  Low-Pass Filter/1 -> [v_pcc_lp]
  [w] -> Scope7/1
  [i_pcc] -> Scope11/1
  [v_pcc] -> Scope4/1
  Gain7/1 -> Measurements/3(i_abc)
  Gain8/1 -> Measurements/2(v_abc)
  CPU/2(w) -> [w]
  [v_pcc] -> CPU/2(v_g)
  [w] -> Gain1/1
  Gain1/1 -> Discrete-Time Integrator1/1
  Discrete-Time Integrator1/1 -> [wt]
  Step1/1 -> Three-Phase Breaker2/1
  Demux2/3 -> Controlled Voltage Source14/1
  Demux2/1 -> Controlled Voltage Source15/1
  Demux2/2 -> Controlled Voltage Source13/1
  [v_c] -> Demux2/1
  Three-Phase V-I Measurement6/1 -> [v_pcc_abc]
  Three-Phase V-I Measurement6/2 -> [i_pcc_abc]
  dq0 to abc/1 -> Gain/1  "m"
  Delay6/1 -> [v_c]
  connections:
  Controlled Voltage Source14/LConn1 -- Ground2/LConn1 -- Controlled Voltage Source15/LConn1 -- Controlled Voltage Source13/LConn1
  Three-Phase Series RLC Branch5/LConn3 -- Three-Phase Breaker2/LConn3
  Three-Phase Breaker2/RConn1 -- Three-Phase V-I Measurement6/LConn1
  Three-Phase Breaker2/RConn2 -- Three-Phase V-I Measurement6/LConn2
  Three-Phase Breaker2/LConn2 -- Three-Phase Series RLC Branch5/LConn2
  Controlled Voltage Source15/RConn1 -- Three-Phase Series RLC Branch5/RConn1
  Three-Phase Series RLC Branch5/LConn1 -- Three-Phase Breaker2/LConn1
  Controlled Voltage Source13/RConn1 -- Three-Phase Series RLC Branch5/RConn2
  Three-Phase Breaker2/RConn3 -- Three-Phase V-I Measurement6/LConn3
  Controlled Voltage Source14/RConn1 -- Three-Phase Series RLC Branch5/RConn3
  A/RConn1 -- Three-Phase V-I Measurement6/RConn1
  Three-Phase V-I Measurement6/RConn2 -- B/RConn1
  C/RConn1 -- Three-Phase V-I Measurement6/RConn3

== system mmc_model/Electrical Model/Variant Subsystem/infinite_bus ==
  Controlled Voltage Source13 : spsControlledVoltageSourceLib/Controlled Voltage Source  Initialize=on  Source_Type=AC  Amplitude=0  Phase=0  Frequency=0  Measurements=None
  Controlled Voltage Source14 : spsControlledVoltageSourceLib/Controlled Voltage Source  Initialize=on  Source_Type=AC  Amplitude=0  Phase=0  Frequency=0  Measurements=None
  Controlled Voltage Source15 : spsControlledVoltageSourceLib/Controlled Voltage Source  Initialize=on  Source_Type=AC  Amplitude=0  Phase=0  Frequency=0  Measurements=None
  Demux2 : Demux  Outputs=3
  Ground2 : spsGroundLib/Ground  LConnTagsString=a
  Mux : Mux  Inputs=3
  Sine Wave3 : Sin  Amplitude=stiffGrid.vpeak  Frequency=stiffGrid.w  Phase=pi/2  SampleTime=0
  Sine Wave4 : Sin  Amplitude=stiffGrid.vpeak  Frequency=stiffGrid.w  Phase=pi/2-2*pi/3  SampleTime=0
  Sine Wave5 : Sin  Amplitude=stiffGrid.vpeak  Frequency=stiffGrid.w  Phase=pi/2+2*pi/3  SampleTime=0
  Three-Phase Series RLC Branch5 : spsThreePhaseSeriesRLCBranchLib/Three-Phase Series RLC Branch  LConnTagsString=A|B|C  RConnTagsString=A|B|C  BranchType=RL  Resistance=stiffGrid.r_si  Inductance=stiffGrid.l_si  Capacitance=1e-6  Measurements=None
  A : PMIOPort  Side=Left
  B : PMIOPort  Port=2  Side=Left
  C : PMIOPort  Port=3  Side=Left
  wires:
  Mux/1 -> Demux2/1
  Demux2/2 -> Controlled Voltage Source13/1
  Demux2/1 -> Controlled Voltage Source15/1
  Demux2/3 -> Controlled Voltage Source14/1
  Sine Wave5/1 -> Mux/3
  Sine Wave3/1 -> Mux/1
  Sine Wave4/1 -> Mux/2
  connections:
  Controlled Voltage Source13/LConn1 -- Controlled Voltage Source14/LConn1 -- Ground2/LConn1 -- Controlled Voltage Source15/LConn1
  Controlled Voltage Source13/RConn1 -- Three-Phase Series RLC Branch5/RConn2
  Controlled Voltage Source14/RConn1 -- Three-Phase Series RLC Branch5/RConn3
  Controlled Voltage Source15/RConn1 -- Three-Phase Series RLC Branch5/RConn1
  A/RConn1 -- Three-Phase Series RLC Branch5/LConn1
  B/RConn1 -- Three-Phase Series RLC Branch5/LConn2
  Three-Phase Series RLC Branch5/LConn3 -- C/RConn1

== system mmc_model/Electrical Model/Variant Subsystem/short_circuited ==
  Ground1 : spsGroundLib/Ground  LConnTagsString=a
  Three-Phase Series RLC Branch1 : spsThreePhaseSeriesRLCBranchLib/Three-Phase Series RLC Branch  LConnTagsString=A|B|C  RConnTagsString=A|B|C  BranchType=R  Resistance=100  Inductance=load2.l_si  Capacitance=1e-6  Measurements=None
  Three-Phase Series RLC Branch7 : spsThreePhaseSeriesRLCBranchLib/Three-Phase Series RLC Branch  LConnTagsString=A|B|C  RConnTagsString=A|B|C  BranchType=R  Resistance=100  Inductance=load2.l_si  Capacitance=1e-6  Measurements=None
  Three-Phase Breaker1 : spsThreePhaseBreakerLib/Three-Phase Breaker  InitialState=open  SwitchA=on  SwitchB=on  SwitchC=on  SwitchTimes=[1.4]  External=off  BreakerResistance=0.01  SnubberResistance=1e6  SnubberCapacitance=inf  Measurements=None
  A : PMIOPort  Side=Left
  B : PMIOPort  Port=2  Side=Left
  C : PMIOPort  Port=3  Side=Left
  connections:
  A/RConn1 -- Three-Phase Breaker1/LConn1 -- Three-Phase Series RLC Branch7/LConn1
  B/RConn1 -- Three-Phase Breaker1/LConn2 -- Three-Phase Series RLC Branch7/LConn2
  C/RConn1 -- Three-Phase Breaker1/LConn3 -- Three-Phase Series RLC Branch7/LConn3
  Ground1/LConn1 -- Three-Phase Series RLC Branch7/RConn3 -- Three-Phase Series RLC Branch7/RConn2 -- Three-Phase Series RLC Branch1/RConn2 -- Three-Phase Series RLC Branch1/RConn1 -- Three-Phase Series RLC Branch1/RConn3 -- Three-Phase Series RLC Branch7/RConn1
  Three-Phase Breaker1/RConn1 -- Three-Phase Series RLC Branch1/LConn1
  Three-Phase Breaker1/RConn2 -- Three-Phase Series RLC Branch1/LConn2
  Three-Phase Breaker1/RConn3 -- Three-Phase Series RLC Branch1/LConn3

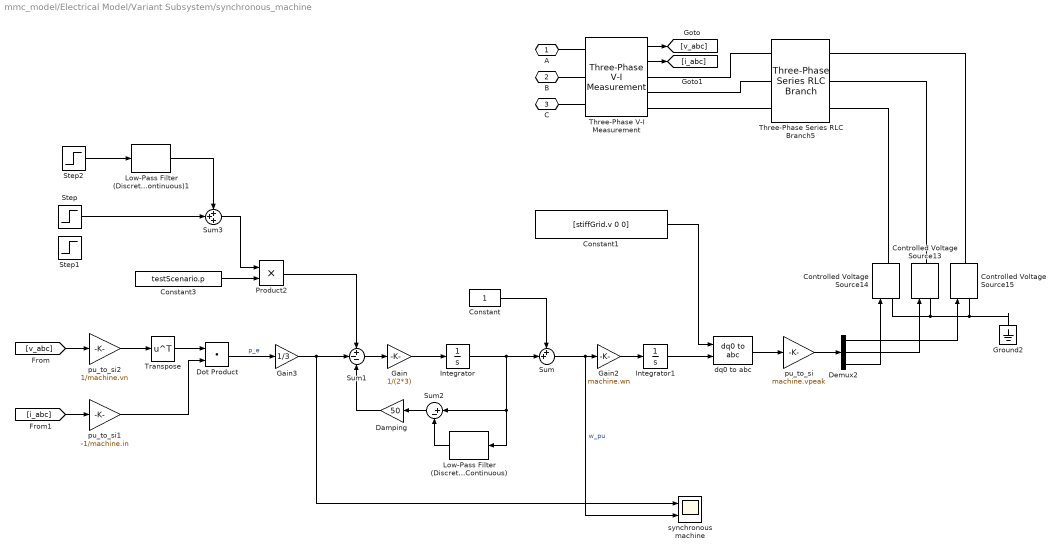
== system mmc_model/Electrical Model/Variant Subsystem/synchronous_machine ==
  Constant : Constant
  Constant1 : Constant  Value=[stiffGrid.v 0 0]
  Constant3 : Constant  Value=testScenario.p
  Controlled Voltage Source13 : spsControlledVoltageSourceLib/Controlled Voltage Source  Initialize=on  Source_Type=AC  Amplitude=0  Phase=0  Frequency=0  Measurements=None
  Controlled Voltage Source14 : spsControlledVoltageSourceLib/Controlled Voltage Source  Initialize=on  Source_Type=AC  Amplitude=0  Phase=0  Frequency=0  Measurements=None
  Controlled Voltage Source15 : spsControlledVoltageSourceLib/Controlled Voltage Source  Initialize=on  Source_Type=AC  Amplitude=0  Phase=0  Frequency=0  Measurements=None
  Damping : Gain  Gain=50
  Demux2 : Demux  Outputs=3
  Dot Product : DotProduct  OutDataTypeStr=Inherit: Inherit via internal rule
  Gain : Gain  Gain=1/(2*3)
  Gain2 : Gain  Gain=machine.wn
  Gain3 : Gain  Gain=1/3
  Ground2 : spsGroundLib/Ground  LConnTagsString=a
  Integrator : Integrator
  Integrator1 : Integrator
  Low-Pass Filter (Discrete or Continuous) : eeGeneralControl/Low-Pass Filter (Discrete or Continuous)  K=1  T=0.1  B=inf  A=-inf  init_option=Inherited from block input  x0=0  Ts=-1
  Low-Pass Filter (Discrete or Continuous)1 : eeGeneralControl/Low-Pass Filter (Discrete or Continuous)  K=1  T=0.1  B=inf  A=-inf  init_option=Inherited from block input  x0=0  Ts=-1
  Product2 : Product
  Step : Step  Time=loadStep.stepDown  After=-1  SampleTime=0
  Step1 : Step  Time=loadStep.stepUp  After=0.8  SampleTime=0
  Step2 : Step  Time=0.3  SampleTime=0
  Sum : Sum  Inputs=++|
  Sum1 : Sum  Inputs=+--
  Sum2 : Sum  Inputs=|+-
  Sum3 : Sum  Inputs=+++
  Three-Phase Series RLC Branch5 : spsThreePhaseSeriesRLCBranchLib/Three-Phase Series RLC Branch  LConnTagsString=A|B|C  RConnTagsString=A|B|C  BranchType=RL  Resistance=machine.tr.r_si  Inductance=machine.tr.l_si  Capacitance=1e-6  Measurements=None
  Three-Phase V-I Measurement : spsThreePhaseVIMeasurementLib/Three-Phase V-I Measurement  VoltageMeasurement=phase-to-ground  SetLabelV=off  LabelV=Vabc  Vpu=off  VpuLL=off  CurrentMeasurement=yes  SetLabelI=off  LabelI=Iabc  Ipu=off  Pbase=100e6  Vbase=500e3  OutputType=Complex  PhasorSimulation=off  PSBequivalent=0
  Transpose : Math  Operator=transpose
  dq0 to abc : spsdq0toabcLib/dq0 to abc  Alignment=Aligned with phase A axis
  pu_to_si : Gain  Gain=machine.vpeak
  pu_to_si1 : Gain  Gain=-1/machine.in
  pu_to_si2 : Gain  Gain=1/machine.vn
  synchronous machine : Scope  NumInputPorts=2
  A : PMIOPort  Side=Left
  B : PMIOPort  Port=2  Side=Left
  C : PMIOPort  Port=3  Side=Left
  wires:
  Demux2/2 -> Controlled Voltage Source13/1
  Demux2/1 -> Controlled Voltage Source15/1
  Demux2/3 -> Controlled Voltage Source14/1
  Transpose/1 -> Dot Product/1
  Dot Product/1 -> Gain3/1  "p_e"
  Gain/1 -> Integrator/1
  Sum1/1 -> Gain/1
  Sum2/1 -> Damping/1
  Low-Pass Filter (Discrete or Continuous)/1 -> Sum2/2
  Constant/1 -> Sum/1
  Sum/1 -> synchronous machine/2, Gain2/1  "w_pu"
  Gain2/1 -> Integrator1/1
  dq0 to abc/1 -> pu_to_si/1
  Integrator1/1 -> dq0 to abc/2
  Constant1/1 -> dq0 to abc/1
  pu_to_si/1 -> Demux2/1
  pu_to_si1/1 -> Dot Product/2
  pu_to_si2/1 -> Transpose/1
  Damping/1 -> Sum1/3
  Three-Phase V-I Measurement/1 -> [v_abc]
  Three-Phase V-I Measurement/2 -> [i_abc]
  [i_abc] -> pu_to_si1/1
  [v_abc] -> pu_to_si2/1
  Gain3/1 -> Sum1/2, synchronous machine/1
  Sum3/1 -> Product2/1
  Constant3/1 -> Product2/2
  Step2/1 -> Low-Pass Filter (Discrete or Continuous)1/1
  Low-Pass Filter (Discrete or Continuous)1/1 -> Sum3/1
  Product2/1 -> Sum1/1
  Integrator/1 -> Sum/2, Sum2/1, Low-Pass Filter (Discrete or Continuous)/1
  Step/1 -> Sum3/2
  connections:
  Ground2/LConn1 -- Controlled Voltage Source15/LConn1 -- Controlled Voltage Source13/LConn1 -- Controlled Voltage Source14/LConn1
  Controlled Voltage Source13/RConn1 -- Three-Phase Series RLC Branch5/RConn2
  Controlled Voltage Source14/RConn1 -- Three-Phase Series RLC Branch5/RConn3
  Controlled Voltage Source15/RConn1 -- Three-Phase Series RLC Branch5/RConn1
  A/RConn1 -- Three-Phase V-I Measurement/LConn1
  B/RConn1 -- Three-Phase V-I Measurement/LConn2
  Three-Phase V-I Measurement/LConn3 -- C/RConn1
  Three-Phase V-I Measurement/RConn1 -- Three-Phase Series RLC Branch5/LConn1
  Three-Phase V-I Measurement/RConn2 -- Three-Phase Series RLC Branch5/LConn2
  Three-Phase V-I Measurement/RConn3 -- Three-Phase Series RLC Branch5/LConn3

== system mmc_model/CPU/Current Limiting Control/Adaptive VI/Subsystem3 ==
  i_dq : Inport
  w : Inport  Port=2
  Gain : Gain  Gain=J  Multiplication=Matrix(K*u) (u vector)
  Gain1 : Gain  Gain=machine.tr.l
  Gain2 : Gain  Gain=machine.tr.r
  Product : Product
  Sum8 : Sum  Inputs=++|
  dm_dq : Outport
  wires:
  Gain1/1 -> Sum8/2
  Sum8/1 -> dm_dq/1  "dm_dq"
  Product/1 -> Gain/1
  Gain/1 -> Gain1/1  "dm_dq"
  w/1 -> Product/1
  i_dq/1 -> Gain2/1, Product/2
  Gain2/1 -> Sum8/1

== system mmc_model/CPU/Current Limiting Control/Adaptive VI/abs ==
  x : Inport
  Dot Product : DotProduct  OutDataTypeStr=Inherit: Inherit via internal rule
  Sqrt3 : Sqrt
  abs : Outport
  wires:
  Sqrt3/1 -> abs/1
  x/1 -> Dot Product/2, Dot Product/1
  Dot Product/1 -> Sqrt3/1

== system mmc_model/CPU/Current Limiting Control/Current Control/abs ==
  x : Inport
  Dot Product : DotProduct  OutDataTypeStr=Inherit: Inherit via internal rule
  Sqrt3 : Sqrt
  abs : Outport
  wires:
  Sqrt3/1 -> abs/1
  x/1 -> Dot Product/2, Dot Product/1
  Dot Product/1 -> Sqrt3/1

== system mmc_model/CPU/Current Limiting Control/Current Limiting Control/SOA_iref ==
  i_ref_dq : Inport
  Constant6 : Constant  Value=clc.i_lim
  Constant7 : Constant  Value=clc.i_lim
  Demux : Demux  Outputs=2
  Gain1 : Gain  Gain=-1
  Gain9 : Gain  Gain=-1
  Mux : Mux  Inputs=2
  Saturation Dynamic1 : simulink/Discontinuities/Saturation Dynamic  OutMin=[]  OutMax=[]  OutDataTypeStr=Inherit: Same as second input  OutDataType=fixdt(1, 16)  OutScaling=2^-10  DoSatur=off
  Saturation Dynamic2 : simulink/Discontinuities/Saturation Dynamic  OutMin=[]  OutMax=[]  OutDataTypeStr=Inherit: Same as second input  OutDataType=fixdt(1, 16)  OutScaling=2^-10  DoSatur=off
  Sqrt3 : Sqrt
  Square1 : Math  Operator=square
  Square4 : Math  Operator=square
  Sum5 : Sum  Inputs=|-+
  i_ref_dq_lim : Outport
  wires:
  Saturation Dynamic1/1 -> Mux/1, Square4/1
  Demux/1 -> Saturation Dynamic1/2
  Square4/1 -> Sum5/1
  Sum5/1 -> Sqrt3/1
  Demux/2 -> Saturation Dynamic2/2
  Sqrt3/1 -> Gain1/1, Saturation Dynamic2/1
  i_ref_dq/1 -> Demux/1
  Saturation Dynamic2/1 -> Mux/2  "i_q_ref_soa"
  Mux/1 -> i_ref_dq_lim/1
  Square1/1 -> Sum5/2
  Constant6/1 -> Square1/1
  Gain9/1 -> Saturation Dynamic1/3
  Constant7/1 -> Saturation Dynamic1/1, Gain9/1
  Gain1/1 -> Saturation Dynamic2/3

== system mmc_model/CPU/Current Limiting Control/Current Limiting Control/Subsystem3 ==
  i_dq : Inport
  w : Inport  Port=2
  Gain : Gain  Gain=J  Multiplication=Matrix(K*u) (u vector)
  Gain1 : Gain  Gain=machine.tr.l
  Gain2 : Gain  Gain=machine.tr.r
  Product : Product
  Sum8 : Sum  Inputs=++|
  dm_dq : Outport
  wires:
  Gain1/1 -> Sum8/2
  Sum8/1 -> dm_dq/1  "dm_dq"
  Product/1 -> Gain/1
  Gain/1 -> Gain1/1  "dm_dq"
  w/1 -> Product/1
  i_dq/1 -> Gain2/1, Product/2
  Gain2/1 -> Sum8/1

== system mmc_model/CPU/Current Limiting Control/Safety Filter/correction ==
  In1 : Inport
  Constant : Constant  Value=0.5
  Constant1 : Constant
  Delay : Delay  DelayLength=1  InitialCondition=0
  Product : Product
  Product1 : Product
  Sum1 : Sum  Inputs=|+-
  Sum2 : Sum  Inputs=++|
  Out1 : Outport
  wires:
  Delay/1 -> Product1/2
  Sum2/1 -> Product/1
  Sum1/1 -> Out1/1
  Product/1 -> Sum1/1
  Constant/1 -> Sum2/2, Product1/1
  In1/1 -> Delay/1, Product/2
  Product1/1 -> Sum1/2
  Constant1/1 -> Sum2/1

== system mmc_model/CPU/GFM Control/EDPC (modified)/Z ==
  i_dq : Inport
  w : Inport  Port=2
  Gain : Gain  Gain=J  Multiplication=Matrix(K*u) (u vector)
  Gain1 : Gain  Gain=machine.tr.l
  Gain2 : Gain  Gain=machine.tr.r
  Product : Product
  Sum8 : Sum  Inputs=++|
  dm_dq : Outport
  wires:
  Gain1/1 -> Sum8/2
  Sum8/1 -> dm_dq/1  "dm_dq"
  Product/1 -> Gain/1
  Gain/1 -> Gain1/1  "dm_dq"
  w/1 -> Product/1
  i_dq/1 -> Gain2/1, Product/2
  Gain2/1 -> Sum8/1

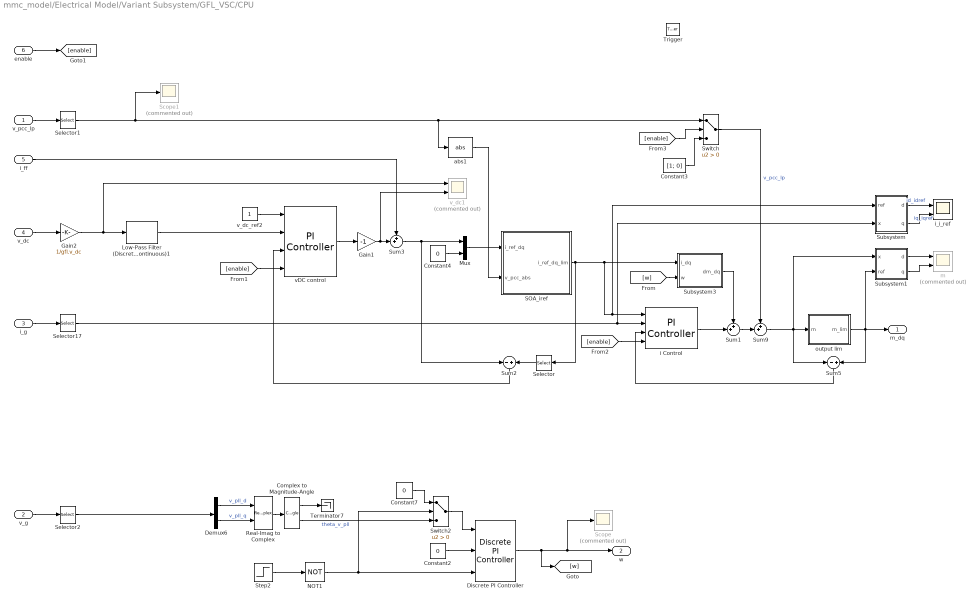
== system mmc_model/Electrical Model/Variant Subsystem/GFL_VSC/CPU ==
  v_pcc_lp : Inport
  v_g : Inport  Port=2
  i_g : Inport  Port=3
  v_dc : Inport  Port=4
  i_ff : Inport  Port=5
  enable : Inport  Port=6
  Trigger : TriggerPort  VariantControl=(inherit)
  Complex to Magnitude-Angle : ComplexToMagnitudeAngle
  Constant2 : Constant  Value=0
  Constant3 : Constant  Value=[1; 0]
  Constant4 : Constant  Value=0
  Constant7 : Constant  Value=0
  Demux6 : Demux  Outputs=2
  Discrete PI Controller : eeDiscretePi/Discrete PI Controller  Kp=ctrl.machine.pll.kp  Ki=ctrl.machine.pll.ti  Kaw=1  x0=ctrl.machine.pll.w0  Ts=-1
      settings: LibrarySourceBlock=ee_sl_lib/General Control/Discrete PI Controller
  Gain1 : Gain  Gain=-1
  Gain2 : Gain  Gain=1/gfl.v_dc
  Low-Pass Filter (Discrete or Continuous)1 : eeGeneralControl/Low-Pass Filter (Discrete or Continuous)  K=1  T=0.1  B=inf  A=-inf  init_option=Inherited from block input  x0=0  Ts=-1
  Mux : Mux  Inputs=2
  NOT1 : Logic  Operator=NOT  IconShape=distinctive  AllPortsSameDT=off  OutDataTypeStr=boolean
  Real-Imag to Complex : RealImagToComplex
  SOA_iref : Subsystem
  Scope : Scope  Commented=on
  Scope1 : Scope  Commented=on
  Selector : Selector  InputPortWidth=2  IndexOptions=Index vector (dialog)  Indices=[1]  OutputSizes=1
  Selector1 : Selector  InputPortWidth=3  IndexOptions=Index vector (dialog)  Indices=[1 2]  OutputSizes=1
  Selector17 : Selector  InputPortWidth=3  IndexOptions=Index vector (dialog)  Indices=[1 2]  OutputSizes=1
  Selector2 : Selector  InputPortWidth=3  IndexOptions=Index vector (dialog)  Indices=[1 2]  OutputSizes=1
  Step2 : Step  Time=gfl.pll_enable
  Subsystem : Subsystem
  Subsystem1 : Subsystem
  Subsystem3 : Subsystem
  Sum1 : Sum  Inputs=++|
  Sum2 : Sum  Inputs=-|+
  Sum3 : Sum  Inputs=++|
  Sum5 : Sum  Inputs=-|+
  Sum9 : Sum  Inputs=++|
  Switch : Switch  Criteria=u2 > Threshold  SaturateOnIntegerOverflow=off  InputSameDT=off
  Switch2 : Switch  Criteria=u2 > Threshold  SaturateOnIntegerOverflow=off  InputSameDT=off
  Terminator7 : Terminator
  abs1 : library/abs  SystemSampleTime=-1  VariantActivationTime=update diagram  AllowFlexibleInterface=on  Latency=0  AutoFrameSizeCalculation=off
  i Control : library/PI Controller  VariantControl=overcurr_ctrl.sel==1  kp=ctrl.machine.ictrl.kp  ti=ctrl.machine.ictrl.ti  Kaw=1000
  i_i_ref : Scope  NumInputPorts=2
  m : Scope  Commented=on  NumInputPorts=2
  output lim : Subsystem
  vDC control : library/PI Controller  VariantControl=overcurr_ctrl.sel==1  kp=gfl.vdc.kp  ti=1000  Kaw=1
  v_dc1 : Scope  Commented=on  NumInputPorts=2
  v_dc_ref2 : Constant
  m_dq : Outport
  w : Outport  Port=2
  wires:
  i_g/1 -> Selector17/1
  Switch/1 -> Sum9/1  "v_pcc_lp"
  Sum1/1 -> Sum9/2
  Sum9/1 -> output lim/1(m), Sum5/1, Subsystem1/1(x)
  [w] -> Subsystem3/2(w)
  v_pcc_lp/1 -> Selector1/1
  Constant3/1 -> Switch/3
  Sum5/1 -> i Control/3
  Subsystem/1(d) -> i_i_ref/1  "id_idref"
  Subsystem/2(q) -> i_i_ref/2  "iq_iqref"
  Subsystem1/2(q) -> m/2
  Subsystem1/1(d) -> m/1
  output lim/1(m_lim) -> Subsystem1/2(ref), m_dq/1, Sum5/2
  i Control/1 -> Sum1/2
  Selector17/1 -> i Control/2, Subsystem/2(x)
  Selector1/1 -> Scope1/1, abs1/1, Switch/1
  Constant2/1 -> Discrete PI Controller/2
  Discrete PI Controller/1 -> [w], Scope/1, w/1
  NOT1/1 -> Switch2/2, Discrete PI Controller/3
  Real-Imag to Complex/1 -> Complex to Magnitude-Angle/1
  Constant7/1 -> Switch2/1
  Step2/1 -> NOT1/1
  Complex to Magnitude-Angle/2 -> Switch2/3  "theta_v_pll"
  Demux6/2 -> Real-Imag to Complex/2  "v_pll_q"
  Complex to Magnitude-Angle/1 -> Terminator7/1
  Demux6/1 -> Real-Imag to Complex/1  "v_pll_d"
  Switch2/1 -> Discrete PI Controller/1
  v_g/1 -> Selector2/1
  Selector2/1 -> Demux6/1
  SOA_iref/1(i_ref_dq_lim) -> i Control/1, Subsystem/1(ref), Subsystem3/1(i_dq), Selector/1
  abs1/1 -> SOA_iref/2(v_pcc_abs)
  v_dc_ref2/1 -> vDC control/1
  v_dc/1 -> Gain2/1
  Constant4/1 -> Mux/2
  Mux/1 -> SOA_iref/1(i_ref_dq)
  enable/1 -> [enable]
  [enable] -> vDC control/4
  [enable] -> i Control/4
  [enable] -> Switch/2
  Subsystem3/1(dm_dq) -> Sum1/1
  Selector/1 -> Sum2/2
  Sum2/1 -> vDC control/3
  Sum3/1 -> Sum2/1, Mux/1
  Gain1/1 -> v_dc1/2, Sum3/2
  i_ff/1 -> Sum3/1
  Gain2/1 -> v_dc1/1, Low-Pass Filter (Discrete or Continuous)1/1
  Low-Pass Filter (Discrete or Continuous)1/1 -> vDC control/2
  vDC control/1 -> Gain1/1
